simulink model "dvoupatrak_15lan"  (R2019b)
settings: Solver=VariableStepAuto  StartTime=0.0  StopTime=sim_time  RelTol=1e-3  AbsTol=1e-3
InitFcn:
  | parameters_dvoupatrak;
values from neighbouring files (symbols this model uses):
  b_d = b_diameter * ones(6,1)    [parameters_dvoupatrak.m]
  b_l = b_length * ones(6,1)    [parameters_dvoupatrak.m]
  b_rho = b_density * ones(6,1)    [parameters_dvoupatrak.m]
  bp = bpi * ones(15,1)    [parameters_dvoupatrak.m]
  bs = c_specific_damping * ones(15,1)    [parameters_dvoupatrak.m]
  kp = kpi * ones(15,1)    [parameters_dvoupatrak.m]
  ks = c_specific_stiffness * ones(15,1)    [parameters_dvoupatrak.m]
  l0_init = cable_length(node_coords, incidence_table(7:end,:))    [parameters_dvoupatrak.m]
  N = node_coords    [parameters_dvoupatrak.m]
  prestress_cab = 0.95    [simulate.m]
  r_mid = 0.15    [parameters_dvoupatrak.m]
  settling_time = 0.5    [simulate.m]
  sim_time = 5    [simulate.m]
  v1 = sqrt(b_length^2 - (xB-xA)^2 - (yB-yA)^2)    [parameters_dvoupatrak.m]
  v2 = sqrt(b_length^2 - (xC-xB)^2 - (yC-yB)^2)    [parameters_dvoupatrak.m]
undefined symbols (not defined in the file or in its folder): X, Y, Z
libraries: nesl_utility x88, sm_lib x70, cstblocks x15, simulink x8
(part 4 of 4)

== system dvoupatrak_15lan/Tensegrity tower/Excitation Subsystem/Cluster of Random Oscillators <0,1>/Rand Oscillator 14 ==
  freq : Inport
  Uniform Random Number : UniformRandomNumber  Minimum=0  Seed=14  SampleTime=0.1
  Varying Lowpass Filter : cstblocks/Linear Parameter Varying/Varying Lowpass Filter  N=2
      settings: SourceProductName=Control System Toolbox
  Out1 : Outport
  wires:
  Varying Lowpass Filter/1 -> Out1/1
  freq/1 -> Varying Lowpass Filter/2
  Uniform Random Number/1 -> Varying Lowpass Filter/1

== system dvoupatrak_15lan/Tensegrity tower/Excitation Subsystem/Cluster of Random Oscillators <0,1>/Rand Oscillator 15 ==
  freq : Inport
  Uniform Random Number : UniformRandomNumber  Minimum=0  Seed=15  SampleTime=0.1
  Varying Lowpass Filter : cstblocks/Linear Parameter Varying/Varying Lowpass Filter  N=2
      settings: SourceProductName=Control System Toolbox
  Out1 : Outport
  wires:
  Uniform Random Number/1 -> Varying Lowpass Filter/1
  freq/1 -> Varying Lowpass Filter/2
  Varying Lowpass Filter/1 -> Out1/1

== system dvoupatrak_15lan/Tensegrity tower/Excitation Subsystem/Cluster of Random Oscillators <0,1>/Rand Oscillator 2 ==
  freq : Inport
  Uniform Random Number : UniformRandomNumber  Minimum=0  Seed=1  SampleTime=0.1
  Varying Lowpass Filter : cstblocks/Linear Parameter Varying/Varying Lowpass Filter  N=2
      settings: SourceProductName=Control System Toolbox
  Out1 : Outport
  wires:
  Varying Lowpass Filter/1 -> Out1/1
  freq/1 -> Varying Lowpass Filter/2
  Uniform Random Number/1 -> Varying Lowpass Filter/1

== system dvoupatrak_15lan/Tensegrity tower/Excitation Subsystem/Cluster of Random Oscillators <0,1>/Rand Oscillator 3 ==
  freq : Inport
  Uniform Random Number : UniformRandomNumber  Minimum=0  Seed=3  SampleTime=0.1
  Varying Lowpass Filter : cstblocks/Linear Parameter Varying/Varying Lowpass Filter  N=2
      settings: SourceProductName=Control System Toolbox
  Out1 : Outport
  wires:
  Uniform Random Number/1 -> Varying Lowpass Filter/1
  freq/1 -> Varying Lowpass Filter/2
  Varying Lowpass Filter/1 -> Out1/1

== system dvoupatrak_15lan/Tensegrity tower/Excitation Subsystem/Cluster of Random Oscillators <0,1>/Rand Oscillator 4 ==
  freq : Inport
  Uniform Random Number : UniformRandomNumber  Minimum=0  Seed=4  SampleTime=0.1
  Varying Lowpass Filter : cstblocks/Linear Parameter Varying/Varying Lowpass Filter  N=2
      settings: SourceProductName=Control System Toolbox
  Out1 : Outport
  wires:
  Varying Lowpass Filter/1 -> Out1/1
  freq/1 -> Varying Lowpass Filter/2
  Uniform Random Number/1 -> Varying Lowpass Filter/1

== system dvoupatrak_15lan/Tensegrity tower/Excitation Subsystem/Cluster of Random Oscillators <0,1>/Rand Oscillator 5 ==
  freq : Inport
  Uniform Random Number : UniformRandomNumber  Minimum=0  Seed=5  SampleTime=0.1
  Varying Lowpass Filter : cstblocks/Linear Parameter Varying/Varying Lowpass Filter  N=2
      settings: SourceProductName=Control System Toolbox
  Out1 : Outport
  wires:
  Uniform Random Number/1 -> Varying Lowpass Filter/1
  freq/1 -> Varying Lowpass Filter/2
  Varying Lowpass Filter/1 -> Out1/1

== system dvoupatrak_15lan/Tensegrity tower/Excitation Subsystem/Cluster of Random Oscillators <0,1>/Rand Oscillator 6 ==
  freq : Inport
  Uniform Random Number : UniformRandomNumber  Minimum=0  Seed=6  SampleTime=0.1
  Varying Lowpass Filter : cstblocks/Linear Parameter Varying/Varying Lowpass Filter  N=2
      settings: SourceProductName=Control System Toolbox
  Out1 : Outport
  wires:
  Varying Lowpass Filter/1 -> Out1/1
  freq/1 -> Varying Lowpass Filter/2
  Uniform Random Number/1 -> Varying Lowpass Filter/1

== system dvoupatrak_15lan/Tensegrity tower/Excitation Subsystem/Cluster of Random Oscillators <0,1>/Rand Oscillator 7 ==
  freq : Inport
  Uniform Random Number : UniformRandomNumber  Minimum=0  Seed=7  SampleTime=0.1
  Varying Lowpass Filter : cstblocks/Linear Parameter Varying/Varying Lowpass Filter  N=2
      settings: SourceProductName=Control System Toolbox
  Out1 : Outport
  wires:
  Uniform Random Number/1 -> Varying Lowpass Filter/1
  freq/1 -> Varying Lowpass Filter/2
  Varying Lowpass Filter/1 -> Out1/1

== system dvoupatrak_15lan/Tensegrity tower/Excitation Subsystem/Cluster of Random Oscillators <0,1>/Rand Oscillator 8 ==
  freq : Inport
  Uniform Random Number : UniformRandomNumber  Minimum=0  Seed=8  SampleTime=0.1
  Varying Lowpass Filter : cstblocks/Linear Parameter Varying/Varying Lowpass Filter  N=2
      settings: SourceProductName=Control System Toolbox
  Out1 : Outport
  wires:
  Varying Lowpass Filter/1 -> Out1/1
  freq/1 -> Varying Lowpass Filter/2
  Uniform Random Number/1 -> Varying Lowpass Filter/1

== system dvoupatrak_15lan/Tensegrity tower/Excitation Subsystem/Cluster of Random Oscillators <0,1>/Rand Oscillator 9 ==
  freq : Inport
  Uniform Random Number : UniformRandomNumber  Minimum=0  Seed=9  SampleTime=0.1
  Varying Lowpass Filter : cstblocks/Linear Parameter Varying/Varying Lowpass Filter  N=2
      settings: SourceProductName=Control System Toolbox
  Out1 : Outport
  wires:
  Uniform Random Number/1 -> Varying Lowpass Filter/1
  freq/1 -> Varying Lowpass Filter/2
  Varying Lowpass Filter/1 -> Out1/1

== matlab function dvoupatrak_15lan/Tensegrity tower/Cables/i-th cable force2/MATLAB Function ==
  data: ks input; ksi output; bs input; l0 input; i input; bsi output; l0i output
function [ksi, bsi, l0i] = params_i(ks, bs, l0, i)

ksi=ks(i);
bsi=bs(i);
l0i=l0(i);

== matlab function dvoupatrak_15lan/Tensegrity tower/Cables/i-th cable force1/MATLAB Function ==
  data: ks input; ksi output; bs input; l0 input; i input; bsi output; l0i output
function [ksi, bsi, l0i] = params_i(ks, bs, l0, i)

ksi=ks(i);
bsi=bs(i);
l0i=l0(i);

== matlab function dvoupatrak_15lan/Tensegrity tower/Cables/i-th cable force2/MATLAB Function1 ==
  data: kp input; Fp output; bp input; l0_init input; dist input; velo input; i input
function Fp = parallel_springs(kp, bp, l0_init, dist, velo, i)

Fpk=kp(i).*(dist-l0_init(i));
Fpb=bp(i).*(velo);
Fp=Fpk+Fpb;
if((dist-l0_init)<=0)
   Fp=0;    
end;

== matlab function dvoupatrak_15lan/Tensegrity tower/Cables/i-th cable force3/MATLAB Function ==
  data: ks input; ksi output; bs input; l0 input; i input; bsi output; l0i output
function [ksi, bsi, l0i] = params_i(ks, bs, l0, i)

ksi=ks(i);
bsi=bs(i);
l0i=l0(i);

== matlab function dvoupatrak_15lan/Tensegrity tower/Cables/i-th cable force3/MATLAB Function1 ==
  data: kp input; Fp output; bp input; l0_init input; dist input; velo input; i input
function Fp = parallel_springs(kp, bp, l0_init, dist, velo, i)

Fpk=kp(i).*(dist-l0_init(i));
Fpb=bp(i).*(velo);
Fp=Fpk+Fpb;
if((dist-l0_init)<=0)
   Fp=0;    
end;

== matlab function dvoupatrak_15lan/Tensegrity tower/Cables/i-th cable force1/MATLAB Function1 ==
  data: kp input; Fp output; bp input; l0_init input; dist input; velo input; i input
function Fp = parallel_springs(kp, bp, l0_init, dist, velo, i)

Fpk=kp(i).*(dist-l0_init(i));
Fpb=bp(i).*(velo);
Fp=Fpk+Fpb;
if((dist-l0_init)<=0)
   Fp=0;    
end;

== matlab function dvoupatrak_15lan/Tensegrity tower/Cables/i-th cable force4/MATLAB Function ==
  data: ks input; ksi output; bs input; l0 input; i input; bsi output; l0i output
function [ksi, bsi, l0i] = params_i(ks, bs, l0, i)

ksi=ks(i);
bsi=bs(i);
l0i=l0(i);

== matlab function dvoupatrak_15lan/Tensegrity tower/Cables/i-th cable force4/MATLAB Function1 ==
  data: kp input; Fp output; bp input; l0_init input; dist input; velo input; i input
function Fp = parallel_springs(kp, bp, l0_init, dist, velo, i)

Fpk=kp(i).*(dist-l0_init(i));
Fpb=bp(i).*(velo);
Fp=Fpk+Fpb;
if((dist-l0_init)<=0)
   Fp=0;    
end;

== matlab function dvoupatrak_15lan/Tensegrity tower/Cables/i-th cable force5/MATLAB Function ==
  data: ks input; ksi output; bs input; l0 input; i input; bsi output; l0i output
function [ksi, bsi, l0i] = params_i(ks, bs, l0, i)

ksi=ks(i);
bsi=bs(i);
l0i=l0(i);

== matlab function dvoupatrak_15lan/Tensegrity tower/Cables/i-th cable force5/MATLAB Function1 ==
  data: kp input; Fp output; bp input; l0_init input; dist input; velo input; i input
function Fp = parallel_springs(kp, bp, l0_init, dist, velo, i)

Fpk=kp(i).*(dist-l0_init(i));
Fpb=bp(i).*(velo);
Fp=Fpk+Fpb;
if((dist-l0_init)<=0)
   Fp=0;    
end;

== matlab function dvoupatrak_15lan/Tensegrity tower/Cables/i-th cable force6/MATLAB Function ==
  data: ks input; ksi output; bs input; l0 input; i input; bsi output; l0i output
function [ksi, bsi, l0i] = params_i(ks, bs, l0, i)

ksi=ks(i);
bsi=bs(i);
l0i=l0(i);

== matlab function dvoupatrak_15lan/Tensegrity tower/Cables/i-th cable force6/MATLAB Function1 ==
  data: kp input; Fp output; bp input; l0_init input; dist input; velo input; i input
function Fp = parallel_springs(kp, bp, l0_init, dist, velo, i)

Fpk=kp(i).*(dist-l0_init(i));
Fpb=bp(i).*(velo);
Fp=Fpk+Fpb;
if((dist-l0_init)<=0)
   Fp=0;    
end;

== matlab function dvoupatrak_15lan/Tensegrity tower/Cables/i-th cable force7/MATLAB Function ==
  data: ks input; ksi output; bs input; l0 input; i input; bsi output; l0i output
function [ksi, bsi, l0i] = params_i(ks, bs, l0, i)

ksi=ks(i);
bsi=bs(i);
l0i=l0(i);

== matlab function dvoupatrak_15lan/Tensegrity tower/Cables/i-th cable force7/MATLAB Function1 ==
  data: kp input; Fp output; bp input; l0_init input; dist input; velo input; i input
function Fp = parallel_springs(kp, bp, l0_init, dist, velo, i)

Fpk=kp(i).*(dist-l0_init(i));
Fpb=bp(i).*(velo);
Fp=Fpk+Fpb;
if((dist-l0_init)<=0)
   Fp=0;    
end;

== matlab function dvoupatrak_15lan/Tensegrity tower/Cables/i-th cable force8/MATLAB Function ==
  data: ks input; ksi output; bs input; l0 input; i input; bsi output; l0i output
function [ksi, bsi, l0i] = params_i(ks, bs, l0, i)

ksi=ks(i);
bsi=bs(i);
l0i=l0(i);

== matlab function dvoupatrak_15lan/Tensegrity tower/Cables/i-th cable force8/MATLAB Function1 ==
  data: kp input; Fp output; bp input; l0_init input; dist input; velo input; i input
function Fp = parallel_springs(kp, bp, l0_init, dist, velo, i)

Fpk=kp(i).*(dist-l0_init(i));
Fpb=bp(i).*(velo);
Fp=Fpk+Fpb;
if((dist-l0_init)<=0)
   Fp=0;    
end;

== matlab function dvoupatrak_15lan/Tensegrity tower/Cables/i-th cable force9/MATLAB Function ==
  data: ks input; ksi output; bs input; l0 input; i input; bsi output; l0i output
function [ksi, bsi, l0i] = params_i(ks, bs, l0, i)

ksi=ks(i);
bsi=bs(i);
l0i=l0(i);

== matlab function dvoupatrak_15lan/Tensegrity tower/Cables/i-th cable force9/MATLAB Function1 ==
  data: kp input; Fp output; bp input; l0_init input; dist input; velo input; i input
function Fp = parallel_springs(kp, bp, l0_init, dist, velo, i)

Fpk=kp(i).*(dist-l0_init(i));
Fpb=bp(i).*(velo);
Fp=Fpk+Fpb;
if((dist-l0_init)<=0)
   Fp=0;    
end;

== matlab function dvoupatrak_15lan/Tensegrity tower/Cables/i-th cable force10/MATLAB Function ==
  data: ks input; ksi output; bs input; l0 input; i input; bsi output; l0i output
function [ksi, bsi, l0i] = params_i(ks, bs, l0, i)

ksi=ks(i);
bsi=bs(i);
l0i=l0(i);

== matlab function dvoupatrak_15lan/Tensegrity tower/Cables/i-th cable force10/MATLAB Function1 ==
  data: kp input; Fp output; bp input; l0_init input; dist input; velo input; i input
function Fp = parallel_springs(kp, bp, l0_init, dist, velo, i)

Fpk=kp(i).*(dist-l0_init(i));
Fpb=bp(i).*(velo);
Fp=Fpk+Fpb;
if((dist-l0_init)<=0)
   Fp=0;    
end;

== matlab function dvoupatrak_15lan/Tensegrity tower/Cables/i-th cable force11/MATLAB Function ==
  data: ks input; ksi output; bs input; l0 input; i input; bsi output; l0i output
function [ksi, bsi, l0i] = params_i(ks, bs, l0, i)

ksi=ks(i);
bsi=bs(i);
l0i=l0(i);

== matlab function dvoupatrak_15lan/Tensegrity tower/Cables/i-th cable force11/MATLAB Function1 ==
  data: kp input; Fp output; bp input; l0_init input; dist input; velo input; i input
function Fp = parallel_springs(kp, bp, l0_init, dist, velo, i)

Fpk=kp(i).*(dist-l0_init(i));
Fpb=bp(i).*(velo);
Fp=Fpk+Fpb;
if((dist-l0_init)<=0)
   Fp=0;    
end;

== matlab function dvoupatrak_15lan/Tensegrity tower/Cables/i-th cable force12/MATLAB Function ==
  data: ks input; ksi output; bs input; l0 input; i input; bsi output; l0i output
function [ksi, bsi, l0i] = params_i(ks, bs, l0, i)

ksi=ks(i);
bsi=bs(i);
l0i=l0(i);

== matlab function dvoupatrak_15lan/Tensegrity tower/Cables/i-th cable force12/MATLAB Function1 ==
  data: kp input; Fp output; bp input; l0_init input; dist input; velo input; i input
function Fp = parallel_springs(kp, bp, l0_init, dist, velo, i)

Fpk=kp(i).*(dist-l0_init(i));
Fpb=bp(i).*(velo);
Fp=Fpk+Fpb;
if((dist-l0_init)<=0)
   Fp=0;    
end;

== matlab function dvoupatrak_15lan/Tensegrity tower/Cables/i-th cable force13/MATLAB Function ==
  data: ks input; ksi output; bs input; l0 input; i input; bsi output; l0i output
function [ksi, bsi, l0i] = params_i(ks, bs, l0, i)

ksi=ks(i);
bsi=bs(i);
l0i=l0(i);

== matlab function dvoupatrak_15lan/Tensegrity tower/Cables/i-th cable force13/MATLAB Function1 ==
  data: kp input; Fp output; bp input; l0_init input; dist input; velo input; i input
function Fp = parallel_springs(kp, bp, l0_init, dist, velo, i)

Fpk=kp(i).*(dist-l0_init(i));
Fpb=bp(i).*(velo);
Fp=Fpk+Fpb;
if((dist-l0_init)<=0)
   Fp=0;    
end;

== matlab function dvoupatrak_15lan/Tensegrity tower/Cables/i-th cable force14/MATLAB Function ==
  data: ks input; ksi output; bs input; l0 input; i input; bsi output; l0i output
function [ksi, bsi, l0i] = params_i(ks, bs, l0, i)

ksi=ks(i);
bsi=bs(i);
l0i=l0(i);

== matlab function dvoupatrak_15lan/Tensegrity tower/Cables/i-th cable force14/MATLAB Function1 ==
  data: kp input; Fp output; bp input; l0_init input; dist input; velo input; i input
function Fp = parallel_springs(kp, bp, l0_init, dist, velo, i)

Fpk=kp(i).*(dist-l0_init(i));
Fpb=bp(i).*(velo);
Fp=Fpk+Fpb;
if((dist-l0_init)<=0)
   Fp=0;    
end;

== matlab function dvoupatrak_15lan/Tensegrity tower/Cables/i-th cable force15/MATLAB Function ==
  data: ks input; ksi output; bs input; l0 input; i input; bsi output; l0i output
function [ksi, bsi, l0i] = params_i(ks, bs, l0, i)

ksi=ks(i);
bsi=bs(i);
l0i=l0(i);

== matlab function dvoupatrak_15lan/Tensegrity tower/Cables/i-th cable force15/MATLAB Function1 ==
  data: kp input; Fp output; bp input; l0_init input; dist input; velo input; i input
function Fp = parallel_springs(kp, bp, l0_init, dist, velo, i)

Fpk=kp(i).*(dist-l0_init(i));
Fpb=bp(i).*(velo);
Fp=Fpk+Fpb;
if((dist-l0_init)<=0)
   Fp=0;    
end;
